simulink model "test_serial"  (R2017b)
settings: Solver=VariableStepAuto  StartTime=0.0  StopTime=9999  FixedStep=0.005  RelTol=1e-3  EnableMultiTasking=on
values from neighbouring files (symbols this model uses):
  A = [1 -dt;0 1]    [kalman_filter.m]    (also in simulink_parameters.m)
  acc_x_gain = 0.975    [simulink_parameters.m]
  acc_x_offset = 0.004    [simulink_parameters.m]
  acc_y_gain = 0.99    [simulink_parameters.m]
  acc_y_offset = 0    [simulink_parameters.m]
  acc_z_gain = 0.97    [simulink_parameters.m]
  acc_z_offset = 0.021    [simulink_parameters.m]
  B = [dt; 0]    [kalman_filter.m]    (also in simulink_parameters.m)
  C = [1 0]    [kalman_filter.m]    (also in simulink_parameters.m)
  mag_x_gain = 1.17    [simulink_parameters.m]
  mag_x_offset = 3.48    [simulink_parameters.m]
  mag_y_gain = 1.133    [simulink_parameters.m]
  mag_y_offset = -0.162    [simulink_parameters.m]
  mag_z_gain = 1.14    [simulink_parameters.m]
  mag_z_offset = 0.177    [simulink_parameters.m]
  Pk_corr_0 = Q    [simulink_parameters.m]
undefined symbols (not defined in the file or in its folder): serial
libraries: instrumentlib x2, simulink x2, peGeneralControl x1
settings Model: Creator=kuba  LastModifiedBy=Michał
settings DataIOCC: LimitDataPoints=on
settings OptimizationCC: LifeSpan=inf
settings DebuggingCC: AllowSymbolicDim=off  SFUnexpectedBacktrackingDiag=warning  SFNoUnconditionalDefaultTransitionDiag=warning  SFExecutionAtInitializationDiag=none
settings ModelReferenceCC: PropagateSignalLabelsOutOfModel=off
settings CodeAppCC: StateflowObjectComments=on
settings GRTTargetCC: TargetLangStandard=C89/C90 (ANSI)
settings ConfigComp: CovMetricSettings=dw  CovHtmlReporting=on  CovSaveCumulativeToWorkspaceVar=on  CovSaveSingleToWorkspaceVar=on  CovExternalEMLEnable=off

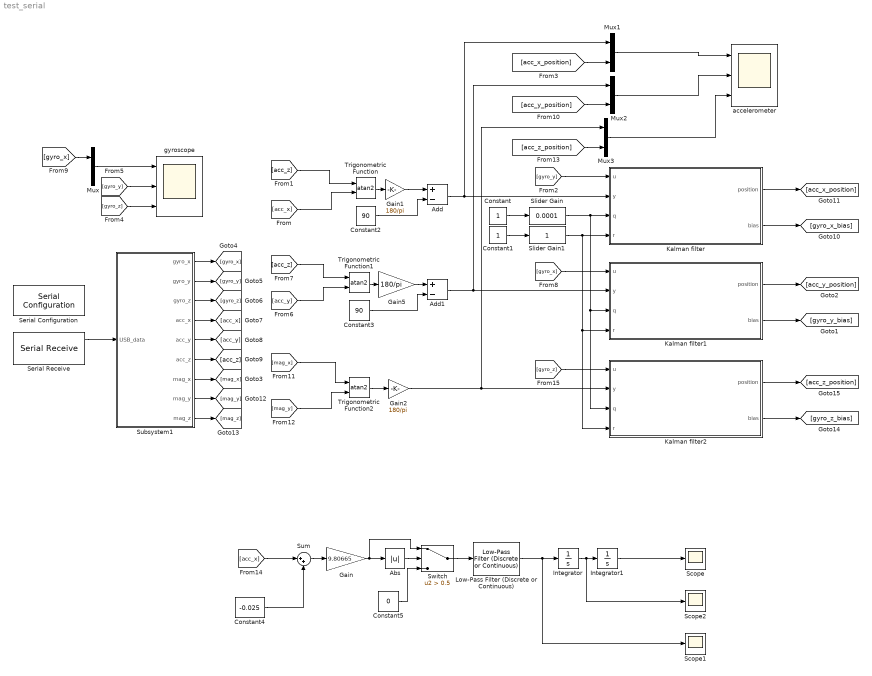
== system test_serial ==
  Abs : Abs
  Add : Sum  Inputs=+-
  Add1 : Sum  Inputs=+-
  Constant : Constant
  Constant1 : Constant
  Constant2 : Constant  Value=90
  Constant3 : Constant  Value=90
  Constant4 : Constant  Value=-0.025
  Constant5 : Constant  Value=0
  Gain : Gain  Gain=9.80665
  Gain1 : Gain  Gain=180/pi
  Gain2 : Gain  Gain=180/pi
  Gain5 : Gain  Gain=180/pi
  Integrator : Integrator
  Integrator1 : Integrator
  Kalman filter : MATLAB Function  TreatAsAtomicUnit=on
  Kalman filter1 : MATLAB Function  TreatAsAtomicUnit=on
  Kalman filter2 : MATLAB Function  TreatAsAtomicUnit=on
  Low-Pass Filter (Discrete or Continuous) : peGeneralControl/Low-Pass Filter (Discrete or Continuous)  K=1  T=1  B=inf  A=-inf  Ts=-1
  Mux{,1..3} (4 alike) : Mux  Inputs=2
  Scope : Scope
  Scope1 : Scope
  Scope2 : Scope
  Serial Configuration : instrumentlib/Serial Configuration  Priority=-200000  ComPortMenu=<Please select a port...>  ComPort=COM4  ObjConstructor=serial('COM4');  BaudRate=9600  DataBits=8  Parity=none  StopBits=1  FlowControl=none  Timeout=10  ByteOrder=LittleEndian
  Serial Receive : instrumentlib/Serial Receive  ComPortMenu=<Please select a port...>  ComPort=COM4  ObjConstructor=serial('COM4');  Terminator=<none>  DataSize="[18   1]"  DataType=uint8  EnableBlockingMode=off  ActionDataUnavailable=Output last received value  CustomValue=0  SampleTime=0.01
  Slider Gain : simulink/Math Operations/Slider Gain  gain=0.0001  low=0  high=1
  Slider Gain1 : simulink/Math Operations/Slider Gain  gain=1  low=0  high=20
  Subsystem1 : Subsystem
  Sum : Sum  Inputs=|++
  Switch : Switch  Criteria=u2 > Threshold  Threshold=0.5
  Trigonometric Function : Trigonometry  Operator=atan2
  Trigonometric Function1 : Trigonometry  Operator=atan2
  Trigonometric Function2 : Trigonometry  Operator=atan2
  "accelerometer " : Scope  NumInputPorts=3
  gyroscope : Scope  NumInputPorts=3
  wires:
  Serial Receive/1 -> Subsystem1/1(USB_data)
  Subsystem1/1(gyro_x) -> [gyro_x]
  Subsystem1/2("gyro_y ") -> [gyro_y]
  Subsystem1/3(gyro_z) -> [gyro_z]
  Subsystem1/4(acc_x) -> [acc_x]
  Subsystem1/5("acc_y ") -> [acc_y]
  Subsystem1/6(acc_z) -> [acc_z]
  [gyro_y] -> Kalman filter/1(u)
  Mux/1 -> gyroscope/1
  [gyro_y] -> gyroscope/2
  [gyro_z] -> gyroscope/3
  [gyro_x] -> Mux/1
  ? -> Mux/2
  Trigonometric Function/1 -> Gain1/1
  [acc_x] -> Trigonometric Function/2
  [acc_z] -> Trigonometric Function/1
  Kalman filter/2(bias) -> [gyro_x_bias]
  Kalman filter/1(position) -> [acc_x_position]
  [gyro_x] -> Kalman filter1/1(u)
  [acc_y] -> Trigonometric Function1/2
  [acc_z] -> Trigonometric Function1/1
  Kalman filter1/2(bias) -> [gyro_y_bias]
  Kalman filter1/1(position) -> [acc_y_position]
  Subsystem1/8(mag_y) -> [mag_y]
  Subsystem1/9(mag_z) -> [mag_z]
  Subsystem1/7(mag_x) -> [mag_x]
  Constant/1 -> Slider Gain/1
  Slider Gain/1 -> Kalman filter2/3(q), Kalman filter1/3(q), Kalman filter/3(q)
  Constant1/1 -> Slider Gain1/1
  Slider Gain1/1 -> Kalman filter/4(r), Kalman filter2/4(r), Kalman filter1/4(r)
  Mux1/1 -> "accelerometer "/1
  Mux2/1 -> "accelerometer "/2
  Add/1 -> Kalman filter/2(y), Mux1/1
  [acc_x_position] -> Mux1/2
  Add1/1 -> Kalman filter1/2(y), Mux2/1
  [acc_y_position] -> Mux2/2
  Constant2/1 -> Add/2
  Trigonometric Function1/1 -> Gain5/1
  Constant3/1 -> Add1/2
  Gain1/1 -> Add/1
  Gain5/1 -> Add1/1
  Kalman filter2/2(bias) -> [gyro_z_bias]
  Kalman filter2/1(position) -> [acc_z_position]
  [mag_x] -> Trigonometric Function2/1
  [mag_y] -> Trigonometric Function2/2
  Trigonometric Function2/1 -> Gain2/1
  Gain2/1 -> Kalman filter2/2(y), Mux3/1
  [gyro_z] -> Kalman filter2/1(u)
  Mux3/1 -> "accelerometer "/3
  [acc_z_position] -> Mux3/2
  Integrator/1 -> Scope2/1, Integrator1/1
  Integrator1/1 -> Scope/1
  [acc_x] -> Sum/1
  Constant4/1 -> Sum/2
  Low-Pass Filter (Discrete or Continuous)/1 -> Integrator/1, Scope1/1
  Switch/1 -> Low-Pass Filter (Discrete or Continuous)/1
  Sum/1 -> Gain/1
  Constant5/1 -> Switch/3
  Gain/1 -> Switch/1, Abs/1
  Abs/1 -> Switch/2

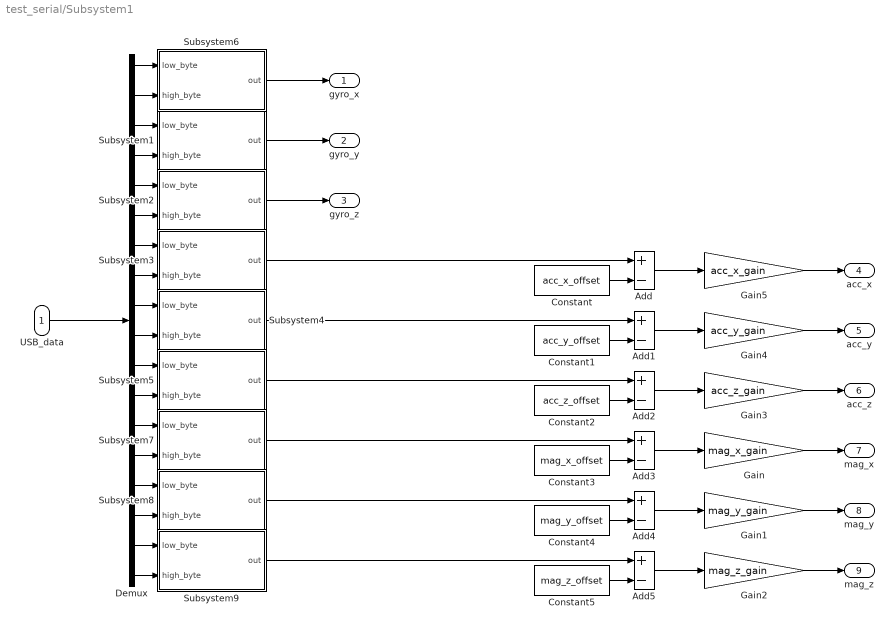
== system test_serial/Subsystem1 ==
  USB_data : Inport
  Add{,1..5} (6 alike) : Sum  Inputs=+-
  Constant : Constant  Value=acc_x_offset
  Constant1 : Constant  Value=acc_y_offset
  Constant2 : Constant  Value=acc_z_offset
  Constant3 : Constant  Value=mag_x_offset
  Constant4 : Constant  Value=mag_y_offset
  Constant5 : Constant  Value=mag_z_offset
  Demux : Demux  Outputs=18
  Gain : Gain  Gain=mag_x_gain
  Gain1 : Gain  Gain=mag_y_gain
  Gain2 : Gain  Gain=mag_z_gain
  Gain3 : Gain  Gain=acc_z_gain
  Gain4 : Gain  Gain=acc_y_gain
  Gain5 : Gain  Gain=acc_x_gain
  Subsystem1 : Subsystem
  Subsystem2 : Subsystem
  Subsystem3 : Subsystem
  Subsystem4 : Subsystem
  Subsystem5 : Subsystem
  Subsystem6 : Subsystem
  Subsystem7 : Subsystem
  Subsystem8 : Subsystem
  Subsystem9 : Subsystem
  gyro_x : Outport
  "gyro_y " : Outport  Port=2
  gyro_z : Outport  Port=3
  acc_x : Outport  Port=4
  "acc_y " : Outport  Port=5
  acc_z : Outport  Port=6
  mag_x : Outport  Port=7
  mag_y : Outport  Port=8
  mag_z : Outport  Port=9
  wires:
  Demux/8 -> Subsystem3/2(high_byte)
  Demux/9 -> Subsystem4/1(low_byte)
  Demux/5 -> Subsystem2/1(low_byte)
  Demux/6 -> Subsystem2/2(high_byte)
  USB_data/1 -> Demux/1
  Demux/7 -> Subsystem3/1(low_byte)
  Demux/12 -> Subsystem5/2(high_byte)
  Demux/11 -> Subsystem5/1(low_byte)
  Demux/10 -> Subsystem4/2(high_byte)
  Demux/3 -> Subsystem1/1(low_byte)
  Demux/4 -> Subsystem1/2(high_byte)
  Demux/1 -> Subsystem6/1(low_byte)
  Demux/2 -> Subsystem6/2(high_byte)
  Subsystem6/1(out) -> gyro_x/1
  Subsystem1/1(out) -> "gyro_y "/1
  Subsystem2/1(out) -> gyro_z/1
  Constant/1 -> Add/2
  Subsystem3/1(out) -> Add/1
  Add/1 -> Gain5/1
  Constant1/1 -> Add1/2
  Subsystem4/1(out) -> Add1/1
  Add1/1 -> Gain4/1
  Constant2/1 -> Add2/2
  Subsystem5/1(out) -> Add2/1
  Add2/1 -> Gain3/1
  Demux/13 -> Subsystem7/1(low_byte)
  Demux/14 -> Subsystem7/2(high_byte)
  Demux/15 -> Subsystem8/1(low_byte)
  Demux/16 -> Subsystem8/2(high_byte)
  Demux/17 -> Subsystem9/1(low_byte)
  Demux/18 -> Subsystem9/2(high_byte)
  Constant3/1 -> Add3/2
  Subsystem7/1(out) -> Add3/1
  Constant4/1 -> Add4/2
  Subsystem8/1(out) -> Add4/1
  Constant5/1 -> Add5/2
  Subsystem9/1(out) -> Add5/1
  Add3/1 -> Gain/1
  Gain/1 -> mag_x/1
  Gain1/1 -> mag_y/1
  Add4/1 -> Gain1/1
  Gain2/1 -> mag_z/1
  Add5/1 -> Gain2/1
  Gain3/1 -> acc_z/1
  Gain4/1 -> "acc_y "/1
  Gain5/1 -> acc_x/1

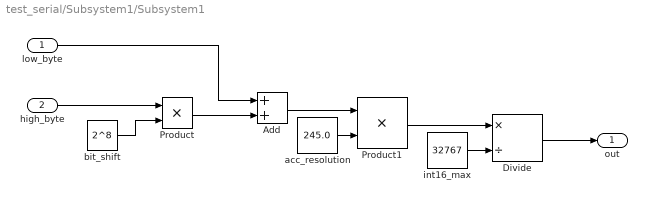
== system test_serial/Subsystem1/Subsystem1 ==
  low_byte : Inport
  high_byte : Inport  Port=2
  Add : Sum  AccumDataTypeStr=int16  OutDataTypeStr=int16
  Divide : Product  Inputs=*/
  Product : Product  OutDataTypeStr=uint16
  Product1 : Product  OutDataTypeStr=double
  acc_resolution : Constant  Value=245.0  OutDataTypeStr=double
  bit_shift : Constant  Value=2^8  OutDataTypeStr=uint16
  int16_max : Constant  Value=32767  OutDataTypeStr=double
  out : Outport  OutDataTypeStr=double
  wires:
  low_byte/1 -> Add/1
  high_byte/1 -> Product/1
  bit_shift/1 -> Product/2
  Product/1 -> Add/2
  acc_resolution/1 -> Product1/2
  Add/1 -> Product1/1
  int16_max/1 -> Divide/2
  Product1/1 -> Divide/1
  Divide/1 -> out/1

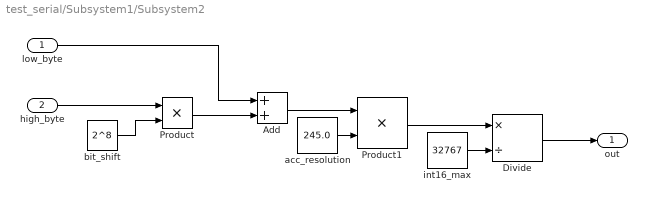
== system test_serial/Subsystem1/Subsystem2 ==
  low_byte : Inport
  high_byte : Inport  Port=2
  Add : Sum  AccumDataTypeStr=int16  OutDataTypeStr=int16
  Divide : Product  Inputs=*/
  Product : Product  OutDataTypeStr=uint16
  Product1 : Product  OutDataTypeStr=double
  acc_resolution : Constant  Value=245.0  OutDataTypeStr=double
  bit_shift : Constant  Value=2^8  OutDataTypeStr=uint16
  int16_max : Constant  Value=32767  OutDataTypeStr=double
  out : Outport  OutDataTypeStr=double
  wires:
  low_byte/1 -> Add/1
  high_byte/1 -> Product/1
  bit_shift/1 -> Product/2
  Product/1 -> Add/2
  acc_resolution/1 -> Product1/2
  Add/1 -> Product1/1
  int16_max/1 -> Divide/2
  Product1/1 -> Divide/1
  Divide/1 -> out/1

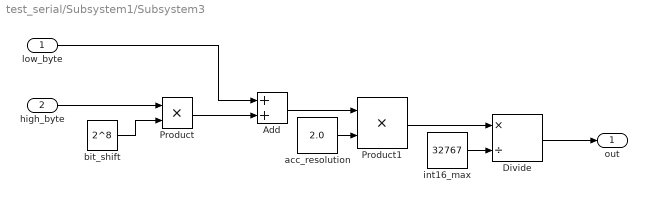
== system test_serial/Subsystem1/Subsystem3 ==
  low_byte : Inport
  high_byte : Inport  Port=2
  Add : Sum  AccumDataTypeStr=int16  OutDataTypeStr=int16
  Divide : Product  Inputs=*/
  Product : Product  OutDataTypeStr=uint16
  Product1 : Product  OutDataTypeStr=double
  acc_resolution : Constant  Value=2.0  OutDataTypeStr=double
  bit_shift : Constant  Value=2^8  OutDataTypeStr=uint16
  int16_max : Constant  Value=32767  OutDataTypeStr=double
  out : Outport  OutDataTypeStr=double
  wires:
  low_byte/1 -> Add/1
  high_byte/1 -> Product/1
  bit_shift/1 -> Product/2
  Product/1 -> Add/2
  acc_resolution/1 -> Product1/2
  Add/1 -> Product1/1
  int16_max/1 -> Divide/2
  Product1/1 -> Divide/1
  Divide/1 -> out/1

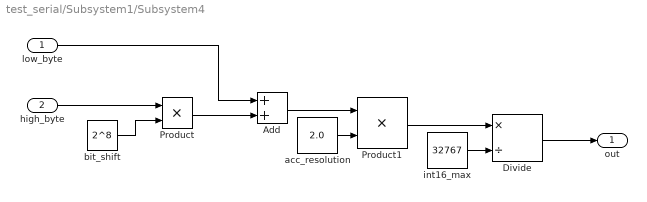
== system test_serial/Subsystem1/Subsystem4 ==
  low_byte : Inport
  high_byte : Inport  Port=2
  Add : Sum  AccumDataTypeStr=int16  OutDataTypeStr=int16
  Divide : Product  Inputs=*/
  Product : Product  OutDataTypeStr=uint16
  Product1 : Product  OutDataTypeStr=double
  acc_resolution : Constant  Value=2.0  OutDataTypeStr=double
  bit_shift : Constant  Value=2^8  OutDataTypeStr=uint16
  int16_max : Constant  Value=32767  OutDataTypeStr=double
  out : Outport  OutDataTypeStr=double
  wires:
  low_byte/1 -> Add/1
  high_byte/1 -> Product/1
  bit_shift/1 -> Product/2
  Product/1 -> Add/2
  acc_resolution/1 -> Product1/2
  Add/1 -> Product1/1
  int16_max/1 -> Divide/2
  Product1/1 -> Divide/1
  Divide/1 -> out/1

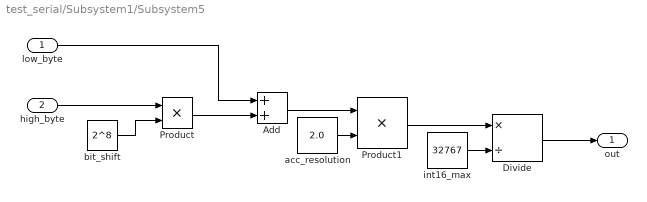
== system test_serial/Subsystem1/Subsystem5 ==
  low_byte : Inport
  high_byte : Inport  Port=2
  Add : Sum  AccumDataTypeStr=int16  OutDataTypeStr=int16
  Divide : Product  Inputs=*/
  Product : Product  OutDataTypeStr=uint16
  Product1 : Product  OutDataTypeStr=double
  acc_resolution : Constant  Value=2.0  OutDataTypeStr=double
  bit_shift : Constant  Value=2^8  OutDataTypeStr=uint16
  int16_max : Constant  Value=32767  OutDataTypeStr=double
  out : Outport  OutDataTypeStr=double
  wires:
  low_byte/1 -> Add/1
  high_byte/1 -> Product/1
  bit_shift/1 -> Product/2
  Product/1 -> Add/2
  acc_resolution/1 -> Product1/2
  Add/1 -> Product1/1
  int16_max/1 -> Divide/2
  Product1/1 -> Divide/1
  Divide/1 -> out/1

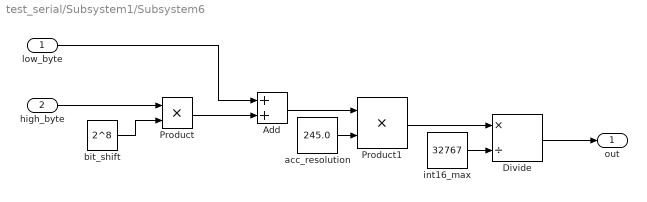
== system test_serial/Subsystem1/Subsystem6 ==
  low_byte : Inport
  high_byte : Inport  Port=2
  Add : Sum  AccumDataTypeStr=int16  OutDataTypeStr=int16
  Divide : Product  Inputs=*/
  Product : Product  OutDataTypeStr=uint16
  Product1 : Product  OutDataTypeStr=double
  acc_resolution : Constant  Value=245.0  OutDataTypeStr=double
  bit_shift : Constant  Value=2^8  OutDataTypeStr=uint16
  int16_max : Constant  Value=32767  OutDataTypeStr=double
  out : Outport  OutDataTypeStr=double
  wires:
  low_byte/1 -> Add/1
  high_byte/1 -> Product/1
  bit_shift/1 -> Product/2
  Product/1 -> Add/2
  acc_resolution/1 -> Product1/2
  Add/1 -> Product1/1
  int16_max/1 -> Divide/2
  Product1/1 -> Divide/1
  Divide/1 -> out/1

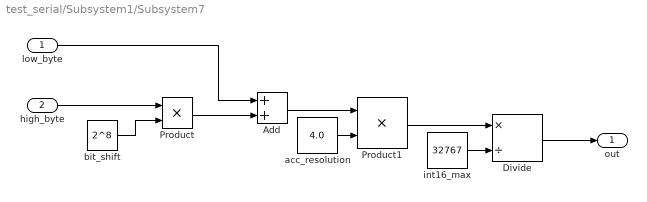
== system test_serial/Subsystem1/Subsystem7 ==
  low_byte : Inport
  high_byte : Inport  Port=2
  Add : Sum  AccumDataTypeStr=int16  OutDataTypeStr=int16
  Divide : Product  Inputs=*/
  Product : Product  OutDataTypeStr=uint16
  Product1 : Product  OutDataTypeStr=double
  acc_resolution : Constant  Value=4.0  OutDataTypeStr=double
  bit_shift : Constant  Value=2^8  OutDataTypeStr=uint16
  int16_max : Constant  Value=32767  OutDataTypeStr=double
  out : Outport  OutDataTypeStr=double
  wires:
  low_byte/1 -> Add/1
  high_byte/1 -> Product/1
  bit_shift/1 -> Product/2
  Product/1 -> Add/2
  acc_resolution/1 -> Product1/2
  Add/1 -> Product1/1
  int16_max/1 -> Divide/2
  Product1/1 -> Divide/1
  Divide/1 -> out/1

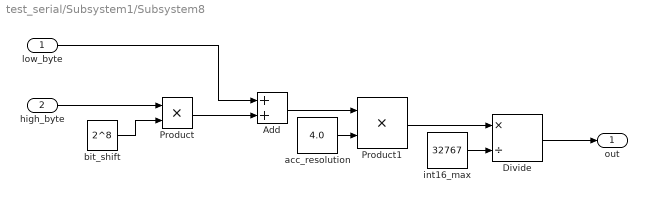
== system test_serial/Subsystem1/Subsystem8 ==
  low_byte : Inport
  high_byte : Inport  Port=2
  Add : Sum  AccumDataTypeStr=int16  OutDataTypeStr=int16
  Divide : Product  Inputs=*/
  Product : Product  OutDataTypeStr=uint16
  Product1 : Product  OutDataTypeStr=double
  acc_resolution : Constant  Value=4.0  OutDataTypeStr=double
  bit_shift : Constant  Value=2^8  OutDataTypeStr=uint16
  int16_max : Constant  Value=32767  OutDataTypeStr=double
  out : Outport  OutDataTypeStr=double
  wires:
  low_byte/1 -> Add/1
  high_byte/1 -> Product/1
  bit_shift/1 -> Product/2
  Product/1 -> Add/2
  acc_resolution/1 -> Product1/2
  Add/1 -> Product1/1
  int16_max/1 -> Divide/2
  Product1/1 -> Divide/1
  Divide/1 -> out/1

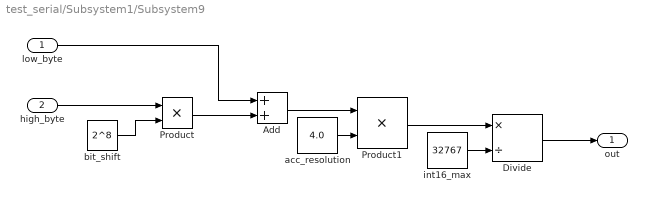
== system test_serial/Subsystem1/Subsystem9 ==
  low_byte : Inport
  high_byte : Inport  Port=2
  Add : Sum  AccumDataTypeStr=int16  OutDataTypeStr=int16
  Divide : Product  Inputs=*/
  Product : Product  OutDataTypeStr=uint16
  Product1 : Product  OutDataTypeStr=double
  acc_resolution : Constant  Value=4.0  OutDataTypeStr=double
  bit_shift : Constant  Value=2^8  OutDataTypeStr=uint16
  int16_max : Constant  Value=32767  OutDataTypeStr=double
  out : Outport  OutDataTypeStr=double
  wires:
  low_byte/1 -> Add/1
  high_byte/1 -> Product/1
  bit_shift/1 -> Product/2
  Product/1 -> Add/2
  acc_resolution/1 -> Product1/2
  Add/1 -> Product1/1
  int16_max/1 -> Divide/2
  Product1/1 -> Divide/1
  Divide/1 -> out/1

== matlab function test_serial/Kalman filter1 ==
  data: u input; position output; y input; Pk_corr_0 parameter; A parameter; B parameter; C parameter; bias output; q input; r input
function [position, bias]  = fcn(u, y, Pk_corr_0, A, B, C, q, r)
    % gyro - u
    % acc  - y 
    Q = [1 0;0 1]*q;   % niepewność procesu (szumy procesowe i niepewność modelowania)
    R = r;             % niepewność pomiaru (im mniejsze tym bardziej ufamy pomiarom)
    persistent xk_corr;
    persistent Pk_corr;
    
    if isempty(Pk_corr)
        Pk_corr = Pk_corr_0;
    end
    
    if isempty(xk_corr)
        xk_corr = [y; 0];
    else
        xk_pred = A*xk_corr + B*u;
        Pk_pred = A*Pk_corr*transpose(A) + Q; 
        error = y - C*xk_pred;
        K = (Pk_pred*transpose(C))/(C*Pk_pred*transpose(C)+R);
        xk_corr = xk_pred + K*error;
        Pk_corr = (eye(2) - K*C)*Pk_pred;
    end
    position = xk_corr(1);
    bias=xk_corr(2);
end

== matlab function test_serial/Kalman filter ==
  data: u input; position output; y input; Pk_corr_0 parameter; A parameter; B parameter; C parameter; bias output; q input; r input
function [position, bias]  = fcn(u, y, Pk_corr_0, A, B, C, q, r)
    % gyro - u
    % acc  - y 
    Q = [1 0;0 1]*q;   % niepewność procesu (szumy procesowe i niepewność modelowania)
    R = r;             % niepewność pomiaru (im mniejsze tym bardziej ufamy pomiarom)
    persistent xk_corr;
    persistent Pk_corr;
    
    if isempty(Pk_corr)
        Pk_corr = Pk_corr_0;
    end
    
    if isempty(xk_corr)
        xk_corr = [y; 0];
    else
        xk_pred = A*xk_corr + B*u;
        Pk_pred = A*Pk_corr*transpose(A) + Q; 
        error = y - C*xk_pred;
        K = (Pk_pred*transpose(C))/(C*Pk_pred*transpose(C)+R);
        xk_corr = xk_pred + K*error;
        Pk_corr = (eye(2) - K*C)*Pk_pred;
    end
    position = xk_corr(1);
    bias=xk_corr(2);
end

== matlab function test_serial/Kalman filter2 ==
  data: u input; position output; y input; Pk_corr_0 parameter; A parameter; B parameter; C parameter; bias output; q input; r input
function [position, bias]  = fcn(u, y, Pk_corr_0, A, B, C, q, r)
    % gyro - u
    % acc  - y 
    Q = [1 0;0 1]*q;   % niepewność procesu (szumy procesowe i niepewność modelowania)
    R = r;             % niepewność pomiaru (im mniejsze tym bardziej ufamy pomiarom)
    persistent xk_corr;
    persistent Pk_corr;
    
    if isempty(Pk_corr)
        Pk_corr = Pk_corr_0;
    end
    
    if isempty(xk_corr)
        xk_corr = [y; 0];
    else
        xk_pred = A*xk_corr + B*u;
        Pk_pred = A*Pk_corr*transpose(A) + Q; 
        error = y - C*xk_pred;
        K = (Pk_pred*transpose(C))/(C*Pk_pred*transpose(C)+R);
        xk_corr = xk_pred + K*error;
        Pk_corr = (eye(2) - K*C)*Pk_pred;
    end
    position = xk_corr(1);
    bias=xk_corr(2);
end
